simulink model "InverseClarkTransformationMatrix"  (R2022a)
settings: Solver=VariableStepAuto  StartTime=0.0  StopTime=10.0  RelTol=1e-3
settings Model: Creator=jff_1  LastModifiedBy=jff_1

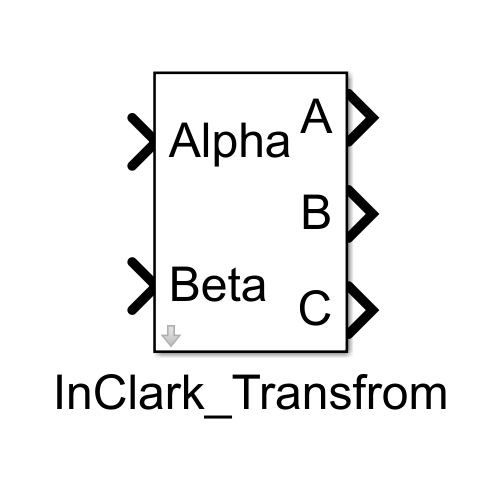
[thumbnail: Simulink's stored preview of the top-level diagram]
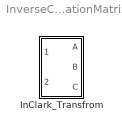
== system InverseClarkTransformationMatrix ==
  InClark_Transfrom : Subsystem
      mask help:
      | 反Clark坐标变换（αβ → abc）
      |
      | 采用幅值不变形式（2/3 系数）
      | 适用于三相对称、无零序分量的系统
      mask Help: 现代永磁同步电机控制原理及MATLAB仿真P6
      mask DialogControl ParameterGroupVar Prompt: 参数
      mask Display:
      | % 输入端口标签（1~3）
      | port_label('input',1,'Alpha');
      | port_label('input',2,'Beta');
      | 
      | % 输出端口标签（1~2）
      | port_label('output',1,'A');
      | port_label('output',2,'B');
      | port_label('output',3,'C');

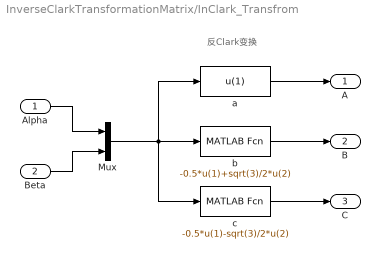
== system InverseClarkTransformationMatrix/InClark_Transfrom ==
  note: 反Clark变换
  Alpha : Inport
  Beta : Inport  Port=2
  Mux : Mux  Inputs=2
  a : MATLABFcn  MATLABFcn=u(1)
  b : MATLABFcn  MATLABFcn=-0.5*u(1)+sqrt(3)/2*u(2)
  c : MATLABFcn  MATLABFcn=-0.5*u(1)-sqrt(3)/2*u(2)
  A : Outport
  B : Outport  Port=2
  C : Outport  Port=3
  wires:
  Beta/1 -> Mux/2
  a/1 -> A/1
  c/1 -> C/1
  Mux/1 -> c/1, b/1, a/1
  b/1 -> B/1
  Alpha/1 -> Mux/1
